simulink model "Heuristic2"  (R2019a)
settings: Solver=ode4  StartTime=0.0  StopTime=100  FixedStep=0.01  MaxStep=0.2  RelTol=1e-3
values from neighbouring files (symbols this model uses):
  operPoint = [x0(i); y0(i); z0(i)]    [Control.m]
  q0 = double(solutions.q0s)    [Control.m]
  q1 = double(solutions.q1s)    [Control.m]
  q2 = double(solutions.q2s)    [Control.m]
  systemD = c2d(system,1)    [Control.m]
settings Model: Creator=Daples  LastModifiedBy=Juan
settings DataIOCC: SaveFormat=Array  SignalLogging=off  DSMLogging=off  ReturnWorkspaceOutputs=off

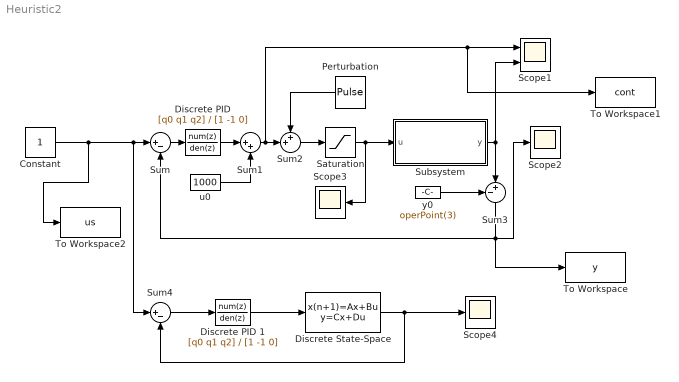
== system Heuristic2 ==
  Constant : Constant
  "Discrete PID " : DiscreteTransferFcn  Numerator=[q0 q1 q2]  Denominator=[1 -1 0]  SampleTime=1
  Discrete PID 1 : DiscreteTransferFcn  Numerator=[q0 q1 q2]  Denominator=[1 -1 0]  SampleTime=1
  Discrete State-Space : DiscreteStateSpace  A=systemD.A  B=systemD.B  C=systemD.C  D=systemD.D
  Perturbation : DiscretePulseGenerator  PulseType=Time based  Amplitude=0.1  Period=10  PulseWidth=5
  Saturation : Saturate  UpperLimit=1500  LowerLimit=0
  Scope1 : Scope  NumInputPorts=2
  Scope2 : Scope
  Scope3 : Scope
  Scope4 : Scope
  Subsystem : Subsystem  mask{Ra=500, Rb=7500, Rc=17.5439, RCs=1, ci=operPoint}
      mask prompts: Ra "Resistance a"; Rb "Resistance b"; Rc "Resistance c"; RCs "Time speed (RC)"; ci "Initial Conditions"
      mask init:
      | x10 = ci(1);
      | x20 = ci(2);
      | y0 = ci(3);
      mask Display: disp("Rössler Attractor")
  Sum : Sum  Inputs=|+-
  Sum1 : Sum  Inputs=|++
  Sum2 : Sum  Inputs=++|
  Sum3 : Sum  Inputs=-+|
  Sum4 : Sum  Inputs=|+-
  To Workspace : ToWorkspace  VariableName=y  SampleTime=-1
  To Workspace1 : ToWorkspace  VariableName=cont  SampleTime=0.01
  To Workspace2 : ToWorkspace  VariableName=us  SampleTime=-1
  "u0 " : Constant  Value=1000
  y0 : Constant  Value=operPoint(3)
  wires:
  Saturation/1 -> Scope3/1, Subsystem/1(u)
  Constant/1 -> To Workspace2/1, Sum4/1, Sum/1
  "u0 "/1 -> Sum1/2
  Sum1/1 -> To Workspace1/1, Scope1/1, Sum2/2
  Perturbation/1 -> Sum2/1
  Sum3/1 -> To Workspace/1, Scope2/1, Sum/2
  y0/1 -> Sum3/1
  Subsystem/1("y ") -> Scope1/2, Sum3/2
  Sum2/1 -> Saturation/1
  "Discrete PID "/1 -> Sum1/1
  Sum/1 -> "Discrete PID "/1
  Discrete PID 1/1 -> Discrete State-Space/1
  Sum4/1 -> Discrete PID 1/1
  Discrete State-Space/1 -> Scope4/1, Sum4/2

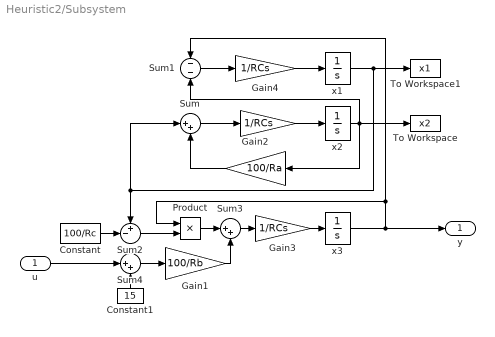
== system Heuristic2/Subsystem ==
  u : Inport
  " " : Gain  Gain=1/RCs
  Constant : Constant  Value=100/Rc
  Constant1 : Constant  Value=15
  Gain1 : Gain  Gain=100/Rb
  Gain2 : Gain  Gain=100/Ra
  Gain3 : Gain  Gain=1/RCs
  Gain4 : Gain  Gain=1/RCs
  Product : Product
  Sum : Sum  Inputs=|++
  Sum1 : Sum  Inputs=--
  Sum2 : Sum  Inputs=+-|
  Sum3 : Sum  Inputs=|++
  Sum4 : Sum  Inputs=|++
  To Workspace : ToWorkspace  VariableName=x2  SampleTime=-1
  To Workspace1 : ToWorkspace  VariableName=x1  SampleTime=-1
  x1 : Integrator  InitialCondition=x10
  x2 : Integrator  InitialCondition=x20
  "x3 " : Integrator  InitialCondition=y0
  "y " : Outport
  wires:
  Sum1/1 -> Gain4/1
  Gain2/1 -> Sum/2
  Sum2/1 -> Product/2
  Product/1 -> Sum3/1
  "x3 "/1 -> "y "/1, Sum1/1, Product/1
  x1/1 -> To Workspace1/1, Sum2/1, Sum/1
  Sum/1 -> " "/1
  Sum3/1 -> Gain3/1
  Constant/1 -> Sum2/2
  x2/1 -> Sum1/2, To Workspace/1, Gain2/1
  u/1 -> Sum4/1
  " "/1 -> x2/1
  Gain3/1 -> "x3 "/1
  Gain4/1 -> x1/1
  Gain1/1 -> Sum3/2
  Constant1/1 -> Sum4/2
  Sum4/1 -> Gain1/1
